simulink model "ball_model_2"  (R2022b)
settings: Solver=VariableStepAuto  StartTime=0.0  StopTime=60.0  RelTol=1e-3
settings Model: Creator=User  LastModifiedBy=User

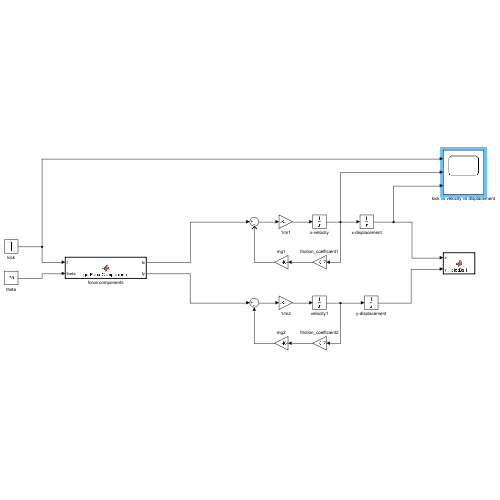
[thumbnail: Simulink's stored preview of the top-level diagram]
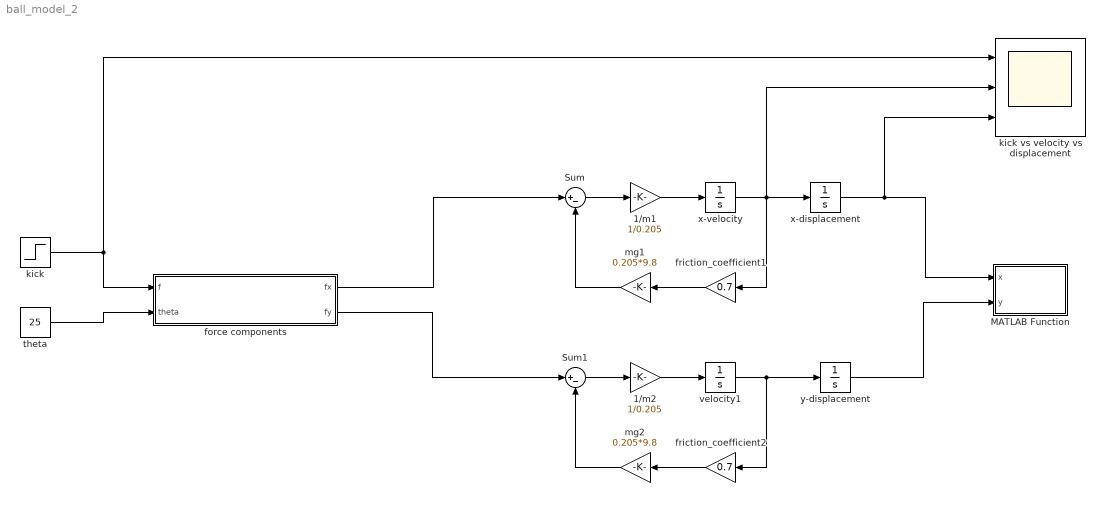
== system ball_model_2 ==
  1/m1 : Gain  Gain=1/0.205
  1/m2 : Gain  Gain=1/0.205
  MATLAB Function : MATLAB Function  TreatAsAtomicUnit=on
  Sum : Sum  Inputs=|+-
  Sum1 : Sum  Inputs=|+-
  force components : MATLAB Function  TreatAsAtomicUnit=on
  friction_coefficient1 : Gain  Gain=0.7
  friction_coefficient2 : Gain  Gain=0.7
  kick : Step  Time=3  Before=3  After=0  SampleTime=0
  kick vs velocity vs displacement : Scope  NumInputPorts=3
  mg1 : Gain  Gain=0.205*9.8
  mg2 : Gain  Gain=0.205*9.8
  theta : Constant  Value=25
  velocity1 : Integrator
  x-displacement : Integrator
  x-velocity : Integrator
  y-displacement : Integrator
  wires:
  force components/1(fx) -> Sum/1
  Sum/1 -> 1/m1/1
  1/m1/1 -> x-velocity/1
  friction_coefficient1/1 -> mg1/1
  mg1/1 -> Sum/2
  x-velocity/1 -> kick vs velocity vs displacement/2, friction_coefficient1/1, x-displacement/1
  velocity1/1 -> friction_coefficient2/1, y-displacement/1
  mg2/1 -> Sum1/2
  1/m2/1 -> velocity1/1
  Sum1/1 -> 1/m2/1
  friction_coefficient2/1 -> mg2/1
  force components/2(fy) -> Sum1/1
  kick/1 -> kick vs velocity vs displacement/1, force components/1(f)
  theta/1 -> force components/2(theta)
  x-displacement/1 -> kick vs velocity vs displacement/3, MATLAB Function/1(x)
  y-displacement/1 -> MATLAB Function/2(y)

== matlab function ball_model_2/force components ==
  data: f input; fx output; theta input; fy output
function [fx,fy] = getForceComponents(f, theta)
    
    fx = f*cos((theta*pi)/180);
    fy = f*sin((theta*pi)/180);

end

== matlab function ball_model_2/MATLAB Function ==
  data: x input; y input
function plotBall(x,y)
    figure(1); clf; hold on; grid on; axis([-30,30,-30,30]);
    plot(x,y,'Color','b','Marker','o');
